simulink model "Q4"  (R2020b)
settings: Solver=VariableStepAuto  StartTime=0.0  StopTime=10.0  RelTol=1e-3
settings Model: Creator=HP  LastModifiedBy=HP

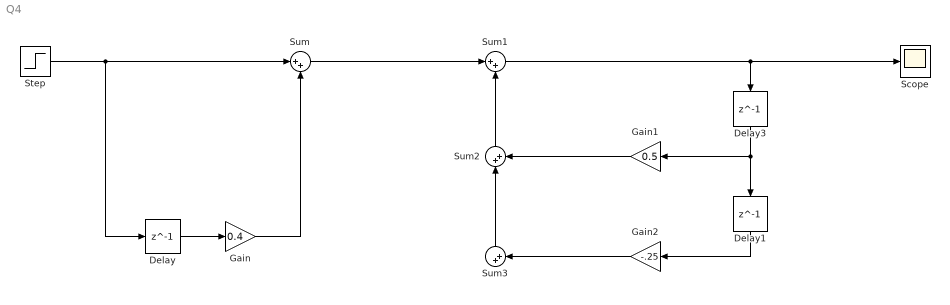
== system Q4 ==
  Delay : Delay  DelayLength=1  InitialCondition=0
  Delay1 : Delay  DelayLength=1  InitialCondition=0
  Delay3 : Delay  DelayLength=1  InitialCondition=0
  Gain : Gain  Gain=0.4
  Gain1 : Gain  Gain=0.5
  Gain2 : Gain  Gain=-.25
  Scope : Scope
  Step : Step  SampleTime=0
  Sum{,1..3} (4 alike) : Sum  Inputs=|++
  wires:
  Step/1 -> Delay/1, Sum/1
  Sum/1 -> Sum1/1
  Gain/1 -> Sum/2
  Sum2/1 -> Sum1/2
  Sum3/1 -> Sum2/1
  Gain1/1 -> Sum2/2
  Gain2/1 -> Sum3/2
  Delay/1 -> Gain/1
  Delay3/1 -> Gain1/1, Delay1/1
  Sum1/1 -> Scope/1, Delay3/1
  Delay1/1 -> Gain2/1
